simulink model "QudaCopter_Model"  (R2025a)
settings: Solver=VariableStepAuto  StartTime=0.0  StopTime=50  RelTol=1e-3
values from neighbouring files (symbols this model uses):
  allocation_matrix = [0   0.5    0.25 0.25 ... (first row only)    [quad_data.m]
  b = data(6)    [quad_data.m]
  d = data(7)    [quad_data.m]
  g = data(5)    [quad_data.m]
  L = data(8)    [quad_data.m]
  m = data(1)    [quad_data.m]
  motors_no = 4    [quad_data.m]
  omega_max = sqrt(2)*omega_nom    [quad_data.m]
  omega_nom = sqrt((m*g)/(motors_no*b))    [quad_data.m]
undefined symbols (not defined in the file or in its folder): sigbuilder_block, Sim3dSensor
libraries: aerolibanim x1, sim3dcameralib x1, sim3dlib x1, uavsim3dlib x1, aerolibobsolete x1, SignalEditorBlockLib x1
settings Model: Creator=Mustafa Taha  LastModifiedBy=Mustafa Taha

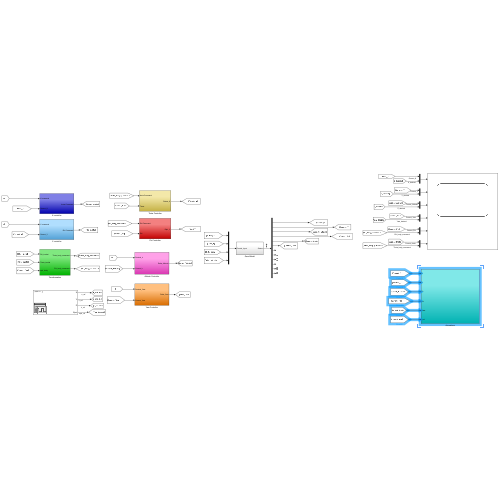
[thumbnail: Simulink's stored preview of the top-level diagram]
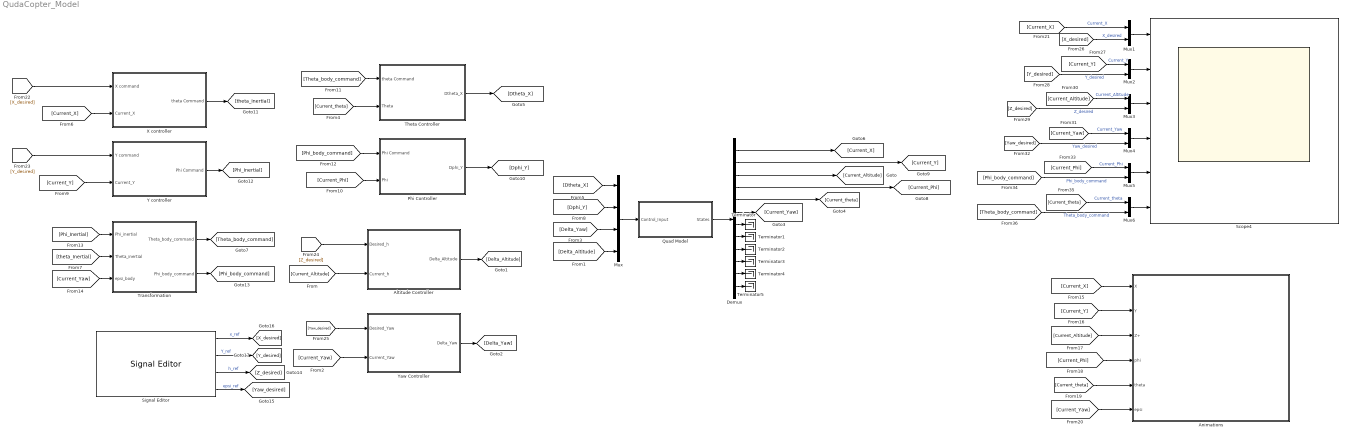
== system QudaCopter_Model ==
  Altitude Controller : Subsystem
  Animations : Subsystem
  Demux : Demux  Outputs=12
  Mux : Mux
  Mux{1..6} (6 alike) : Mux  Inputs=2
  Phi Controller : Subsystem
  Quad Model : Subsystem
  Scope4 : Scope  NumInputPorts=6
      settings: ActiveDisplayYMinimum=-0.62499999999999989  ActiveDisplayYMaximum=5.625  DataLoggingVariableName=ScopeData4
  Signal Editor : SignalEditorBlockLib/Signal Editor  FileName=Quad_path.mat  ActiveScenario=Scenario_1  ActiveSignal=X  IsBus=off  OutputBusObjectStr=Bus: BusObject  SampleTime=0  Interpolate=off  ZeroCross=off  OutputAfterFinalValue=Setting to zero  Unit=inherit  PreserveSignalName=on  ApplySigPropsToAllScenarios=on  ApplySigPropsToAllSignals=off  SignalPropertySource=Dialog parameters
  Terminator{,1..5} (6 alike) : Terminator
  Theta Controller : Subsystem
  Transformation : Subsystem
  X controller : Subsystem
  Y controller : Subsystem
  Yaw Controller : Subsystem
  wires:
  Quad Model/1(States) -> Demux/1
  Mux/1 -> Quad Model/1(Control_Input)
  [Dtheta_X] -> Mux/1
  [Dphi_Y] -> Mux/2
  [Delta_Yaw] -> Mux/3
  Demux/3 -> [Current_Altitude]
  [Current_Altitude] -> Altitude Controller/2(Current_h)
  Altitude Controller/1(Delta_Altitude) -> [Delta_Altitude]
  [Delta_Altitude] -> Mux/4
  [Z_desired] -> Altitude Controller/1(Desired_h)
  [Yaw_desired] -> Yaw Controller/1(Desired_Yaw)
  [Current_Yaw] -> Yaw Controller/2(Current_Yaw)
  Demux/6 -> [Current_Yaw]
  Demux/5 -> [Current_theta]
  Demux/1 -> [Current_X]
  Theta Controller/1(Dtheta_X) -> [Dtheta_X]
  [Current_theta] -> Theta Controller/2(Theta)
  [Theta_body_command] -> Theta Controller/1(theta Command)
  [Current_X] -> X controller/2(Current_X)
  X controller/1(theta Command) -> [theta_Inertial]
  Demux/2 -> [Current_Y]
  Demux/4 -> [Current_Phi]
  [Y_desired] -> Y controller/1(Y command)
  Y controller/1(Phi Command) -> [Phi_Inertial]
  [Current_Y] -> Y controller/2(Current_Y)
  Phi Controller/1(Dphi_Y) -> [Dphi_Y]
  [Current_Phi] -> Phi Controller/2(Phi)
  [Phi_body_command] -> Phi Controller/1(Phi Command)
  [theta_Inertial] -> Transformation/2(Theta_inertial)
  Transformation/1(Theta_body_command) -> [Theta_body_command]
  [Phi_Inertial] -> Transformation/1(Phi_inertial)
  Transformation/2(Phi_body_command) -> [Phi_body_command]
  [Current_Yaw] -> Transformation/3(epsi_body)
  Yaw Controller/1(Delta_Yaw) -> [Delta_Yaw]
  [X_desired] -> X controller/1(X command)
  [Current_X] -> Animations/1(X)
  [Current_Y] -> Animations/2(Y)
  [Current_Altitude] -> Animations/3(Z+)
  [Current_Phi] -> Animations/4(phi)
  [Current_theta] -> Animations/5(theta)
  [Current_Yaw] -> Animations/6(epsi)
  Demux/7 -> Terminator/1
  Demux/8 -> Terminator1/1
  Demux/9 -> Terminator2/1
  Demux/10 -> Terminator3/1
  Demux/11 -> Terminator4/1
  Demux/12 -> Terminator5/1
  [Current_X] -> Mux1/1  "Current_X"
  Signal Editor/2 -> [Y_desired]  "Y_ref"
  Signal Editor/1 -> [X_desired]  "x_ref"
  Signal Editor/3 -> [Z_desired]  "h_ref"
  Signal Editor/4 -> [Yaw_desired]  "epsi_ref"
  [X_desired] -> Mux1/2  "X_desired"
  [Current_Y] -> Mux2/1  "Current_Y"
  [Y_desired] -> Mux2/2  "Y_desired"
  [Current_Altitude] -> Mux3/1  "Current_Altitude"
  [Current_Yaw] -> Mux4/1  "Current_Yaw"
  [Yaw_desired] -> Mux4/2  "Yaw_desired"
  [Current_Phi] -> Mux5/1  "Current_Phi"
  [Phi_body_command] -> Mux5/2  "Phi_body_command"
  [Current_theta] -> Mux6/1  "Current_theta"
  [Theta_body_command] -> Mux6/2  "Theta_body_command"
  Mux1/1 -> Scope4/1
  Mux2/1 -> Scope4/2
  [Z_desired] -> Mux3/2  "Z_desired"
  Mux3/1 -> Scope4/3
  Mux4/1 -> Scope4/4
  Mux5/1 -> Scope4/5
  Mux6/1 -> Scope4/6

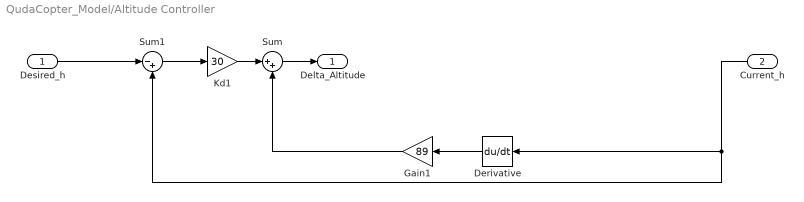
== system QudaCopter_Model/Altitude Controller ==
  Desired_h : Inport
  Current_h : Inport  Port=2
  Derivative : Derivative
  Gain1 : Gain  Gain=89
  Kd1 : Gain  Gain=30
  Sum : Sum  Inputs=|++
  Sum1 : Sum  Inputs=|-+
  Delta_Altitude : Outport
  wires:
  Sum/1 -> Delta_Altitude/1
  Derivative/1 -> Gain1/1
  Desired_h/1 -> Sum1/1
  Kd1/1 -> Sum/1
  Current_h/1 -> Sum1/2, Derivative/1
  Sum1/1 -> Kd1/1
  Gain1/1 -> Sum/2

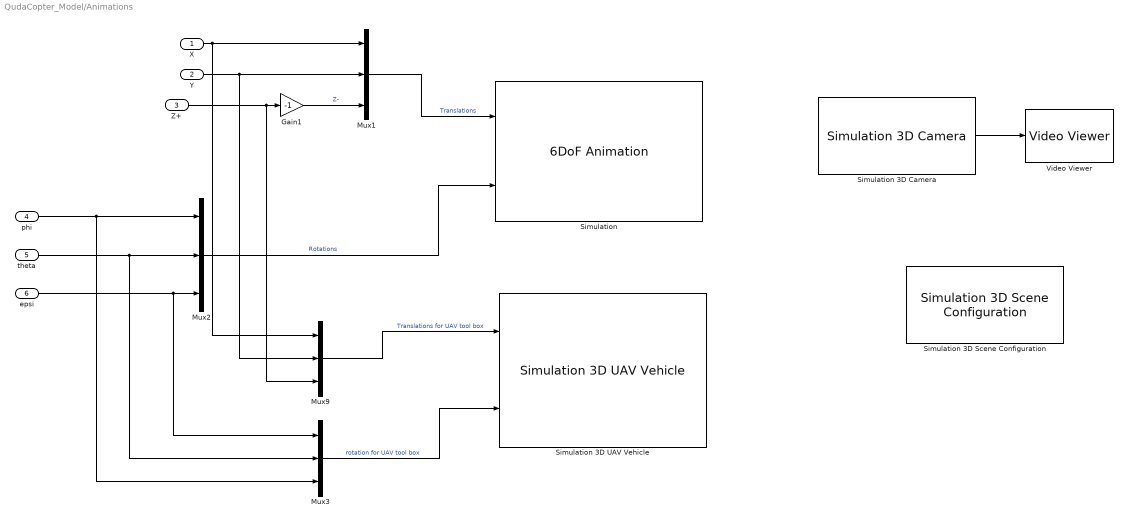
== system QudaCopter_Model/Animations ==
  X : Inport
  Y : Inport  Port=2
  Z+ : Inport  Port=3
  phi : Inport  Port=4
  theta : Inport  Port=5
  epsi : Inport  Port=6
  Gain1 : Gain  Gain=-1
  Mux{1..3,9} (4 alike) : Mux  Inputs=3
  Simulation : aerolibanim/6DoF Animation  u1=[-8 8 -8 8 -6 0]  u2=0.1  u3=1.0  u4=[0 0 0]  u5=Fixed position  u6=[20 50 -20]  u7=10  u8=on
  Simulation 3D Camera : sim3dcameralib/Simulation 3D Camera  Priority=1  sensorTag=Sim3dSensor�  sensorId=1  sensorName=Sim3dSensor�  vehTagList={'Scene Origin'}  vehTag=Scene Origin  CoordinateSystem=ISO8855  mountLoc=Origin  offsetFlag=on  tmountOffset=[0.1, 0, 0]  extTmount=off  rmountOffset=[0, 0, 0]  extRmount=off  FocalLength=[1109, 1109]  OpticalCenter=[640, 360]  ImageSize=[720, 1280]  RadialDistortion=[0, 0]  TangentialDistortion=[0, 0]  SensorSkew=0  VisualizeFieldOfView=off  FieldOfViewRange=61  DepthOutportEnabled=off  SemanticOutportEnabled=off  TransformOutportEnabled=off  SampleTime=-1  mountPoint=[0.1 0 0]  mountOrientation=[0 0 0]  aMode=4  ID=1
      settings: LibrarySourceBlock=uavsim3dlib/Simulation 3D Camera
  Simulation 3D Scene Configuration : sim3dlib/Simulation 3D Scene Configuration  Priority=0  ProjectFormat=Default Scenes  SceneDesc=US city block  ProjectName=C:\Program Files\MATLAB\R2025a\toolbox\shared\sim3d_projects\automotive_project_windows\UE\WindowsNoEditor\VehicleSimulation.exe  ScenePath=/Game/Maps/USCityBlock  EnableOpenDRIVE=off  vehTagList={'Scene Origin'}  vehTag=Scene Origin  AttachedCameraRelativeTranslation=[0 0 0]  FreeCameraDefaultInitialTranslation=[-6, 0, 2]  AttachedCameraRelativeRotation=[0 0 0]  FreeCameraDefaultInitialRotation=[0, -15, 0]  ViewpointName=Custom  FreeCameraInitialTranslation=[0, 0, 0]  ViewpointTranslation=[0 0 0]  FreeCameraInitialRotation=[0, 0, 0]  ViewpointRotation=[0 0 0]  OpVisEn=off  Ts=0.1  EnableWindow=on  EnableRemoteAccess=off  EnableWeather=off  SunAzimuth=90  SunAltitude=40.0  EnableGeospatialSun=off  Latitude=0  Longitude=0  Date=2023-01-01  Time=10:30:00  GeoTimeZone=-5.0  SunDaylightSaving=off  wind=1  clouds=10  EnableVolumetricClouds=off  CloudCoverage=0  CloudAltitude=6  fog=0  rain=0  RaindropsEffect=off  SnowDensity=0  EnableGeospatial=off  TilesetSource=Earth terrain  UseTrueOrigin=off  OriginHeight=200  OriginLatitude=40.744652  OriginLongitude=-73.988864  MapStyle=Aerial  AdditionalAssetIDs=[]  UseAdvancedSunSky=off  SolarTime=11  TimeZone=-5  Day=21  Month=9  Year=2022  UseDaylightSavingTime=on  DSTStartDay=10  DSTStartMonth=3  DSTEndDay=3  DSTEndMonth=11  DSTSwitchHour=2  sensorTag=MainCamera1  sensorId=1  sensorName=MainCamera1  mountLoc=Origin  offsetFlag=off  tmountOffset=[0, 0, 0]  rmountOffset=[0, 0, 0]  HorizontalResolution=1280  VerticalResolution=720  HorizontalFOV=60  mountPoint=[0 0 0]  mountOrientation=[0 0 0]  aMode=4  ID=1  GeoTrigger=Inactive  ViewNameList={'Custom'}  ViewTranslationList={'[0 0 0]'}  ViewRotationList={'[0 0 0]'}
      settings: LibrarySourceBlock=uavsim3dlib/Simulation 3D Scene Configuration
  Simulation 3D UAV Vehicle : uavsim3dlib/Simulation 3D UAV Vehicle  Priority=-1  Mesh=Quadrotor  MeshPath=/MathWorksUAVContent/UAVs/HexaRotorUAV/HexaRotor.HexaRotor  Color=Black  ActorName=SimulinkVehicle1  UseGlobalFrame=off  InitialTranslation=[0 0 0]  InitialRotation=[0 0 0]  InitialTranslationGlobal=[0 0 0]  InitialGeoOrigin=[0 0 0]  InitialRotationGlobal=[0 0 0]  SampleTime=0.1  ActorType=SimulinkVehicle  ID=1  aMode=4  ActorTag=SimulinkVehicle1
  Video Viewer : VideoViewer  FigPos=[803 436 418 304]
  wires:
  Mux2/1 -> Simulation/2  "Rotations"
  X/1 -> Mux1/1, Mux9/1
  Gain1/1 -> Mux1/3  "Z-"
  Z+/1 -> Gain1/1, Mux9/3
  Mux9/1 -> Simulation 3D UAV Vehicle/1  "Translations for UAV tool box"
  Mux1/1 -> Simulation/1  "Translations"
  Y/1 -> Mux1/2, Mux9/2
  phi/1 -> Mux2/1, Mux3/3
  theta/1 -> Mux2/2, Mux3/2
  epsi/1 -> Mux2/3, Mux3/1
  Mux3/1 -> Simulation 3D UAV Vehicle/2  "rotation for UAV tool box"
  Simulation 3D Camera/1 -> Video Viewer/1

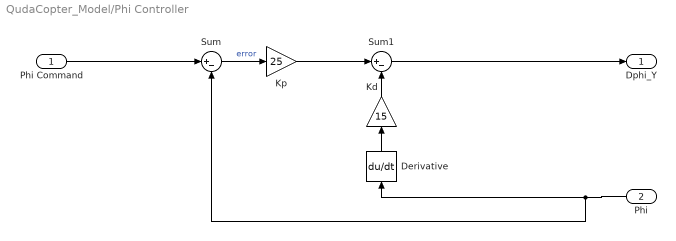
== system QudaCopter_Model/Phi Controller ==
  Phi Command : Inport
  Phi : Inport  Port=2
  Derivative : Derivative
  Kd : Gain  Gain=15
  Kp : Gain  Gain=25
  Sum : Sum  Inputs=|+-
  Sum1 : Sum  Inputs=|+-
  Dphi_Y : Outport
  wires:
  Phi/1 -> Derivative/1, Sum/2
  Sum1/1 -> Dphi_Y/1
  Phi Command/1 -> Sum/1
  Kd/1 -> Sum1/2
  Sum/1 -> Kp/1  "error"
  Kp/1 -> Sum1/1
  Derivative/1 -> Kd/1

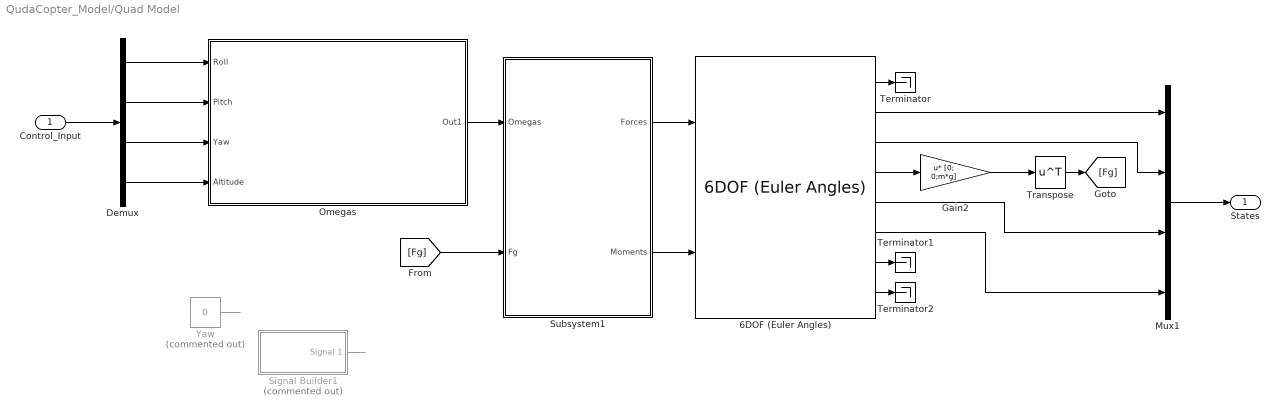
== system QudaCopter_Model/Quad Model ==
  Control_Input : Inport
  6DOF (Euler Angles) : aerolibobsolete/6DOF (Euler Angles)  units=Metric (MKS)  mtype=Fixed  rep=Euler Angles  xme_0=[0 0 -1]  Vm_0=[0 0 0]  eul_0=[0 0 0]  pm_0=[0 0 0]  mass_0=m  mass_e=0.5  mass_f=2.0  inertia=I  inertia_e=eye(3)  inertia_f=2*eye(3)  k_quat=1.0  vre_flag=on  abi_flag=off  aMode=0  xme_statename=''  Vm_statename=''  eul_statename=''  quat_statename=''  pm_statename=''  mass_statename=''
  Demux : Demux
  Gain2 : Gain  Gain=[0; 0;m*g]  Multiplication=Matrix(u*K)
  Mux1 : Mux
  Omegas : Subsystem
  Signal Builder1 : Subsystem  Tag=STV Subsys  Commented=on  LoadFcn=sigbuilder_block('load');  StartFcn=sigbuilder_block('start');  StopFcn=sigbuilder_block('stop');  ClipboardFcn=sigbuilder_block('clipboard');  mask(Sigbuilder block){tuvar=[0:10]}
      mask help: Simulink:masks:SigbuilderBlock_MD
      mask init:
      | if ~strcmp(get_param(bdroot(gcbh),'SimulationStatus'),'stopped') tuvar = sigbuilder_block('maskInit'); end
      settings: CopyFcn=sigbuilder_block('copy');  DeleteFcn=sigbuilder_block('delete');  ModelCloseFcn=sigbuilder_block('modelClose');  PreSaveFcn=sigbuilder_block('preSave');  PauseFcn=sigbuilder_block('pause');  ContinueFcn=sigbuilder_block('continue');  NameChangeFcn=sigbuilder_block('namechange');  OpenFcn=sigbuilder_block('open',[394.2 60 550.8 400.2 ]);  CloseFcn=sigbuilder_block('close');
      mask Display: plot(0, 0, 100, 100,[2, 2, 32, 32, 2], [68, 8, 8, 68, 68],[32, 2], [38, 38], [32, 19, 2],[53, 60, 44], [32, 17, 17, 2],[16, 16, 31, 31]);txt = getActiveGroup(gcbh);text(2, 100, txt,'verticalAlignment', 'top');
  Subsystem1 : Subsystem
  Terminator : Terminator
  Terminator1 : Terminator
  Terminator2 : Terminator
  Transpose : Math  Operator=transpose
  Yaw : Constant  Commented=on  Value=0
  States : Outport
  wires:
  Gain2/1 -> Transpose/1
  Transpose/1 -> [Fg]
  6DOF (Euler Angles)/4 -> Gain2/1
  Subsystem1/2(Moments) -> 6DOF (Euler Angles)/2
  Demux/2 -> Omegas/2("Pitch ")
  Mux1/1 -> States/1
  Demux/4 -> Omegas/4("Altitude ")
  Omegas/1(Out1) -> Subsystem1/1(Omegas)
  Demux/3 -> Omegas/3("Yaw ")
  Subsystem1/1(Forces) -> 6DOF (Euler Angles)/1
  [Fg] -> Subsystem1/2(Fg)
  Yaw/1 -> ?
  Signal Builder1/1(Signal 1) -> ?
  Demux/1 -> Omegas/1("Roll ")
  6DOF (Euler Angles)/6 -> Mux1/4
  6DOF (Euler Angles)/5 -> Mux1/3
  6DOF (Euler Angles)/2 -> Mux1/1
  6DOF (Euler Angles)/3 -> Mux1/2
  Control_Input/1 -> Demux/1
  6DOF (Euler Angles)/1 -> Terminator/1
  6DOF (Euler Angles)/7 -> Terminator1/1
  6DOF (Euler Angles)/8 -> Terminator2/1

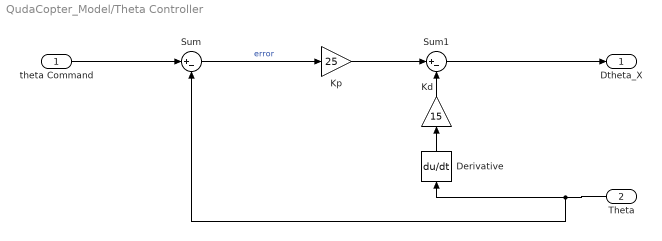
== system QudaCopter_Model/Theta Controller ==
  theta Command : Inport
  Theta : Inport  Port=2
  Derivative : Derivative
  Kd : Gain  Gain=15
  Kp : Gain  Gain=25
  Sum : Sum  Inputs=|+-
  Sum1 : Sum  Inputs=|+-
  Dtheta_X : Outport
  wires:
  Theta/1 -> Derivative/1, Sum/2
  Sum1/1 -> Dtheta_X/1
  theta Command/1 -> Sum/1
  Kd/1 -> Sum1/2
  Sum/1 -> Kp/1  "error"
  Kp/1 -> Sum1/1
  Derivative/1 -> Kd/1

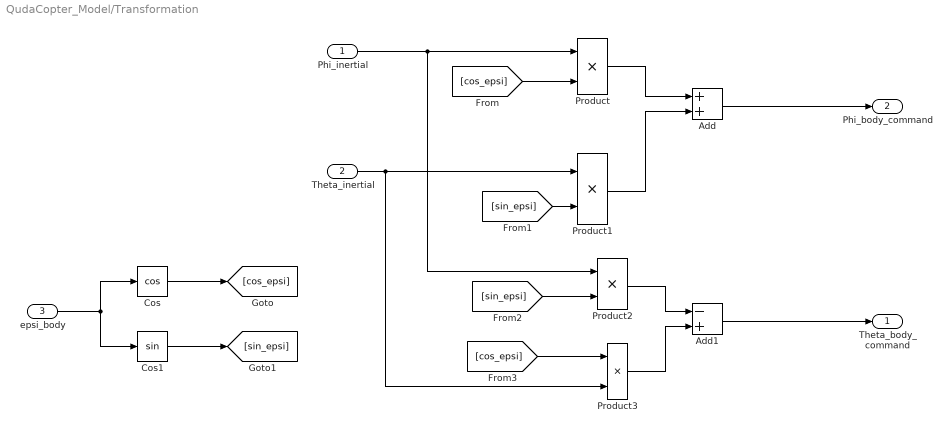
== system QudaCopter_Model/Transformation ==
  Phi_inertial : Inport
  Theta_inertial : Inport  Port=2
  epsi_body : Inport  Port=3
  Add : Sum
  Add1 : Sum  Inputs=-+
  Cos : Trigonometry  Operator=cos
  Cos1 : Trigonometry
  Product{,1..3} (4 alike) : Product
  Theta_body_command : Outport
  Phi_body_command : Outport  Port=2
  wires:
  Phi_inertial/1 -> Product2/1, Product/1
  epsi_body/1 -> Cos1/1, Cos/1
  Cos/1 -> [cos_epsi]
  Theta_inertial/1 -> Product3/2, Product1/1
  Cos1/1 -> [sin_epsi]
  Product/1 -> Add/1
  Product1/1 -> Add/2
  [cos_epsi] -> Product/2
  [sin_epsi] -> Product1/2
  Add/1 -> Phi_body_command/1
  Product3/1 -> Add1/2
  Product2/1 -> Add1/1
  [sin_epsi] -> Product2/2
  [cos_epsi] -> Product3/1
  Add1/1 -> Theta_body_command/1

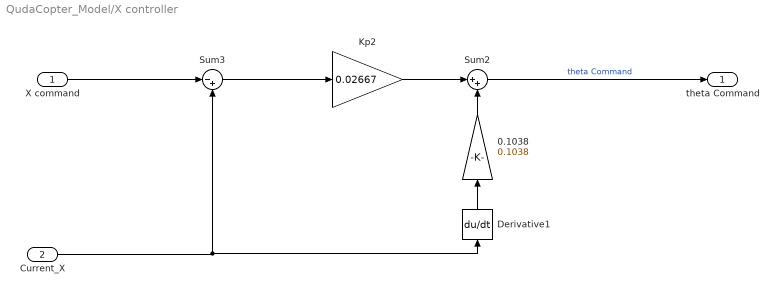
== system QudaCopter_Model/X controller ==
  X command : Inport
  Current_X : Inport  Port=2
  0.1038 : Gain  Gain=0.1038
  Derivative1 : Derivative
  Kp2 : Gain  Gain=0.02667
  Sum2 : Sum  Inputs=|++
  Sum3 : Sum  Inputs=|-+
  theta Command : Outport
  wires:
  Kp2/1 -> Sum2/1
  X command/1 -> Sum3/1
  Sum3/1 -> Kp2/1
  Current_X/1 -> Sum3/2, Derivative1/1
  0.1038/1 -> Sum2/2
  Derivative1/1 -> 0.1038/1
  Sum2/1 -> theta Command/1  "theta Command"

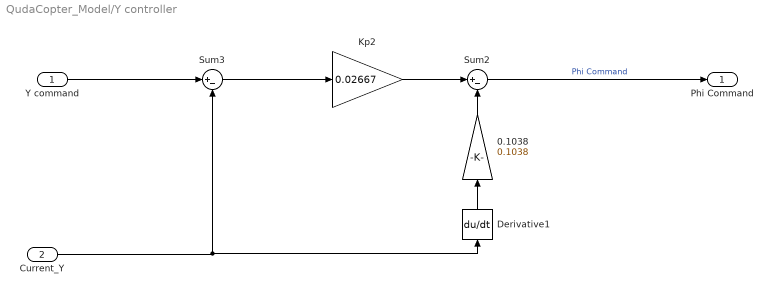
== system QudaCopter_Model/Y controller ==
  Y command : Inport
  Current_Y : Inport  Port=2
  0.1038 : Gain  Gain=0.1038
  Derivative1 : Derivative
  Kp2 : Gain  Gain=0.02667
  Sum2 : Sum  Inputs=|+-
  Sum3 : Sum  Inputs=|+-
  Phi Command : Outport
  wires:
  Kp2/1 -> Sum2/1
  Y command/1 -> Sum3/1
  Sum3/1 -> Kp2/1
  Current_Y/1 -> Sum3/2, Derivative1/1
  0.1038/1 -> Sum2/2
  Derivative1/1 -> 0.1038/1
  Sum2/1 -> Phi Command/1  "Phi Command"

== system QudaCopter_Model/Yaw Controller ==
  Desired_Yaw : Inport
  Current_Yaw : Inport  Port=2
  Derivative : Derivative
  Kd1 : Gain  Gain=304
  Kp : Gain  Gain=322.8
  Sum : Sum  Inputs=|+-
  Sum1 : Sum  Inputs=|+-
  Delta_Yaw : Outport
  wires:
  Sum/1 -> Delta_Yaw/1
  Kp/1 -> Sum/2
  Kd1/1 -> Sum/1
  Current_Yaw/1 -> Sum1/2, Derivative/1
  Sum1/1 -> Kd1/1
  Desired_Yaw/1 -> Sum1/1
  Derivative/1 -> Kp/1

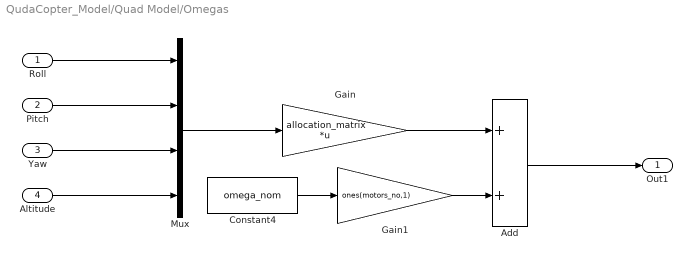
== system QudaCopter_Model/Quad Model/Omegas ==
  "Roll " : Inport
  "Pitch " : Inport  Port=2
  "Yaw " : Inport  Port=3
  "Altitude " : Inport  Port=4
  Add : Sum
  Constant4 : Constant  Value=omega_nom
  Gain : Gain  Gain=allocation_matrix  Multiplication=Matrix(K*u)
  Gain1 : Gain  Gain=ones(motors_no,1)
  Mux : Mux
  Out1 : Outport
  wires:
  Mux/1 -> Gain/1
  "Yaw "/1 -> Mux/3
  Constant4/1 -> Gain1/1
  "Roll "/1 -> Mux/1
  "Pitch "/1 -> Mux/2
  Gain/1 -> Add/1
  "Altitude "/1 -> Mux/4
  Gain1/1 -> Add/2
  Add/1 -> Out1/1

== system QudaCopter_Model/Quad Model/Signal Builder1 ==
  Demux : Demux  Tag=STV Demux  Outputs=1
      settings: DisplayOption=none
  FromWs : FromWorkspace  Tag=STV FromWs  VariableName=tuvar
      SigBuilderData=|
      | common.afterFinalStr = 'Extrapolate'
      | common.sampleTime = 0
      | dataSet.timeRange = [0 10]
      | dataSet.name = 'Group 1'
      | sbobj.Groups.Name = 'Group 1'
      | sbobj.Groups.Signals.Name = 'Signal 1'
      | sbobj.Groups.Signals.XData = [0 4 4 6 6 10]
      | sbobj.Groups.Signals.YData = [0 0.06 5 5 0 0]
  Signal 1 : Outport  Tag=STV Outport
  wires:
  FromWs/1 -> Demux/1
  Demux/1 -> Signal 1/1

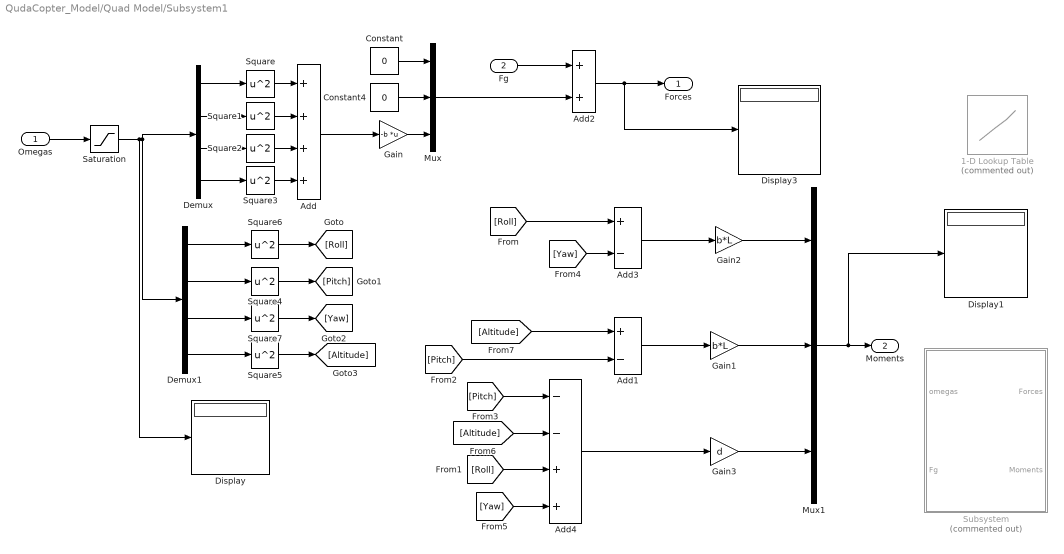
== system QudaCopter_Model/Quad Model/Subsystem1 ==
  Omegas : Inport
  Fg : Inport  Port=2
  1-D Lookup Table : Lookup_n-D  Commented=on  NumberOfTableDimensions=1  BreakpointsForDimension1=[0 omega_nom sqrt(2)*omega_nom]  Table=[-1 0 1]  InternalRulePriority=Speed  RndMeth=Simplest
  Add : Sum  Inputs=++++
  Add1 : Sum  Inputs=+-
  Add2 : Sum
  Add3 : Sum  Inputs=+-
  Add4 : Sum  Inputs=--++
  Constant : Constant  Value=0
  Constant4 : Constant  Value=0
  Demux : Demux
  Demux1 : Demux
  Display : Display
  Display1 : Display
  Display3 : Display
  Gain : Gain  Gain=-b  Multiplication=Matrix(K*u)
  Gain1 : Gain  Gain=b*L
  Gain2 : Gain  Gain=b*L
  Gain3 : Gain  Gain=d
  Mux : Mux  Inputs=3
  Mux1 : Mux  Inputs=3
  Saturation : Saturate  UpperLimit=omega_max
  Square{,1..7} (8 alike) : Math  Operator=square
  Subsystem : Subsystem  Commented=on
  Forces : Outport
  Moments : Outport  Port=2
  wires:
  Add/1 -> Gain/1
  Square2/1 -> Add/3
  Square3/1 -> Add/4
  Square/1 -> Add/1
  Demux/3 -> Square2/1
  Square1/1 -> Add/2
  Demux/2 -> Square1/1
  Fg/1 -> Add2/1
  Mux/1 -> Add2/2
  Demux/4 -> Square3/1
  Gain/1 -> Mux/3
  Add2/1 -> Forces/1, Display3/1
  Demux/1 -> Square/1
  Constant/1 -> Mux/1
  Constant4/1 -> Mux/2
  Demux1/2 -> Square4/1
  Demux1/4 -> Square5/1
  Demux1/1 -> Square6/1
  Demux1/3 -> Square7/1
  Add1/1 -> Gain1/1
  Add3/1 -> Gain2/1
  Add4/1 -> Gain3/1
  Gain2/1 -> Mux1/1
  Gain1/1 -> Mux1/2
  Gain3/1 -> Mux1/3
  Mux1/1 -> Display1/1, Moments/1
  Square6/1 -> [Roll]
  [Roll] -> Add3/1
  [Roll] -> Add4/3
  Square4/1 -> [Pitch]
  [Pitch] -> Add1/2
  [Pitch] -> Add4/1
  [Yaw] -> Add4/4
  [Yaw] -> Add3/2
  Square7/1 -> [Yaw]
  Square5/1 -> [Altitude]
  [Altitude] -> Add4/2
  [Altitude] -> Add1/1
  Saturation/1 -> Demux/1, Demux1/1, Display/1
  Omegas/1 -> Saturation/1

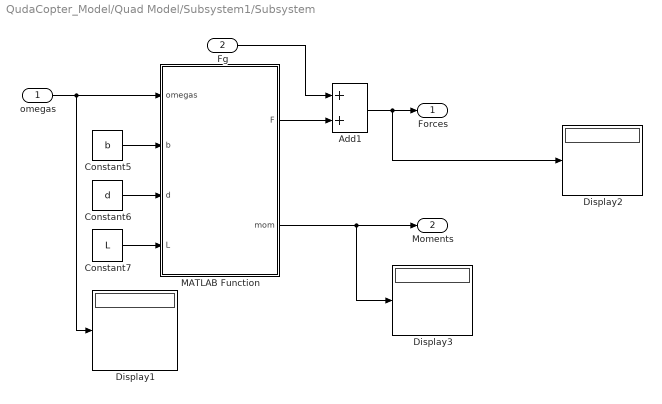
== system QudaCopter_Model/Quad Model/Subsystem1/Subsystem ==
  omegas : Inport
  Fg : Inport  Port=2
  Add1 : Sum
  Constant5 : Constant  Value=b
  Constant6 : Constant  Value=d
  Constant7 : Constant  Value=L
  Display1 : Display
  Display2 : Display
  Display3 : Display
  MATLAB Function : MATLAB Function  TreatAsAtomicUnit=on
  Forces : Outport
  Moments : Outport  Port=2
  wires:
  Constant6/1 -> MATLAB Function/3(d)
  MATLAB Function/1(F) -> Add1/2
  Add1/1 -> Display2/1, Forces/1
  Fg/1 -> Add1/1
  Constant7/1 -> MATLAB Function/4(L)
  Constant5/1 -> MATLAB Function/2(b)
  MATLAB Function/2(mom) -> Display3/1, Moments/1
  omegas/1 -> MATLAB Function/1(omegas), Display1/1

== matlab function QudaCopter_Model/Quad Model/Subsystem1/Subsystem/MATLAB Function ==
  data: omegas input; F output; b input; d input; L input; mom output
function [F,mom] = fcn(omegas,b,d,L)
w1= omegas(1);
w2= omegas(2);
w3= omegas(3);
w4= omegas(4);

%deltas (roll,pitch,yaw,thrust)
F = [0 0 -b*(w1^2 + w2^2 +w3^2 + w4^2)];
mom = [b*L*(w4^2-w2^2)...
    b*L*(w1^2-w3^2)...
    d*(-w2^2-w4^2+w1^2+w3^2)];
